simulink model "NMPC"  (R2017b)
settings: Solver=ode1  StartTime=0.0  StopTime=parSim.Tsim  FixedStep=0.001  RelTol=1e-3  EnableMultiTasking=on
values from neighbouring files (symbols this model uses):
  sysD_Delay = ss(A_Delay,B_Delay,C_Delay,D_Delay,parNMPC.Ts)    [main_GW02.m]
undefined symbols (not defined in the file or in its folder): parNMPC, parSim
libraries: simulink x1
settings Model: Creator=shaen  LastModifiedBy=severine

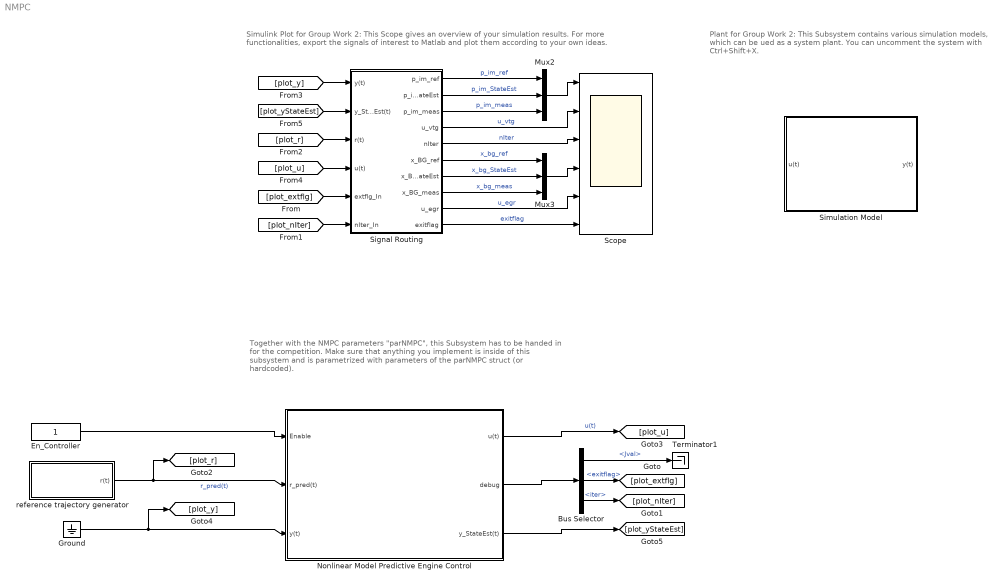
== system NMPC ==
  note: Plant for Group Work 2: This Subsystem contains various
      | simulation models, which can be ued as a system plant. You
      | can uncomment the system with Ctrl+Shift+X.
  note: Together with the NMPC parameters "parNMPC", this Subsystem
      | has to be handed in for the competition. Make sure that
      | anything you implement is inside of this subsystem and is
      | parametrized with parameters of the parNMPC struct (or
      | hardcoded).
  note: Simulink Plot for Group Work 2: This Scope gives an overview of your simulation results.
      | For more functionalities, export the signals of interest to Matlab and plot them according to your
      | own ideas.
  Bus Selector : BusSelector  OutputSignals=Jval,exitflag,iter
  En_Controller : Constant  OutDataTypeStr=boolean
  Ground : Ground
  Mux2 : Mux  Inputs=3
  Mux3 : Mux  Inputs=3
  Nonlinear Model Predictive Engine Control : Subsystem  Description=test
  Scope : Scope  NumInputPorts=6
  Signal Routing : Subsystem
  Simulation Model : Subsystem
  Terminator1 : Terminator
  reference trajectory generator : Subsystem  mask{N=parNMPC.N, Ts=parNMPC.Ts}
      mask prompts: N "NMPC Horizon"; Ts "NMPC Time Step"
      mask DialogControl DescGroupVar Prompt: Reference Generator
      mask DialogControl DescTextVar Prompt: Derivation of the reference vecotrs for every time step for a non-causal NMPC approach.
  wires:
  Signal Routing/10(exitflag) -> Scope/6  "exitflag"
  Mux3/1 -> Scope/4
  Nonlinear Model Predictive Engine Control/2(debug) -> Bus Selector/1
  [plot_r] -> Signal Routing/3(r(t))
  Signal Routing/5(nIter) -> Scope/3  "nIter"
  Signal Routing/4(u_vtg) -> Scope/2  "u_vtg"
  [plot_u] -> Signal Routing/4(u(t))
  Signal Routing/8(x_BG_meas) -> Mux3/3  "x_bg_meas"
  Signal Routing/6(x_BG_ref) -> Mux3/1  "x_bg_ref"
  Mux2/1 -> Scope/1
  Signal Routing/1(p_im_ref) -> Mux2/1  "p_im_ref"
  Bus Selector/3 -> [plot_nIter]  "<iter>"
  reference trajectory generator/1(r(t)) -> [plot_r], Nonlinear Model Predictive Engine Control/2(r_pred(t))  "r_pred(t)"
  Nonlinear Model Predictive Engine Control/1(u(t)) -> [plot_u]  "u(t)"
  Signal Routing/3(p_im_meas) -> Mux2/3  "p_im_meas"
  [plot_y] -> Signal Routing/1(y(t))
  [plot_extflg] -> Signal Routing/5(extflg_In)
  Signal Routing/9(u_egr) -> Scope/5  "u_egr"
  Bus Selector/1 -> Terminator1/1  "<Jval>"
  [plot_nIter] -> Signal Routing/6(nIter_In)
  Bus Selector/2 -> [plot_extflg]  "<exitflag>"
  Nonlinear Model Predictive Engine Control/3(y_StateEst(t)) -> [plot_yStateEst]
  [plot_yStateEst] -> Signal Routing/2(y_StateEst(t))
  Signal Routing/7(x_BG_StateEst) -> Mux3/2  "x_bg_StateEst"
  Signal Routing/2(p_im_StateEst) -> Mux2/2  "p_im_StateEst"
  En_Controller/1 -> Nonlinear Model Predictive Engine Control/1(Enable)
  Ground/1 -> [plot_y], Nonlinear Model Predictive Engine Control/3(y(t))

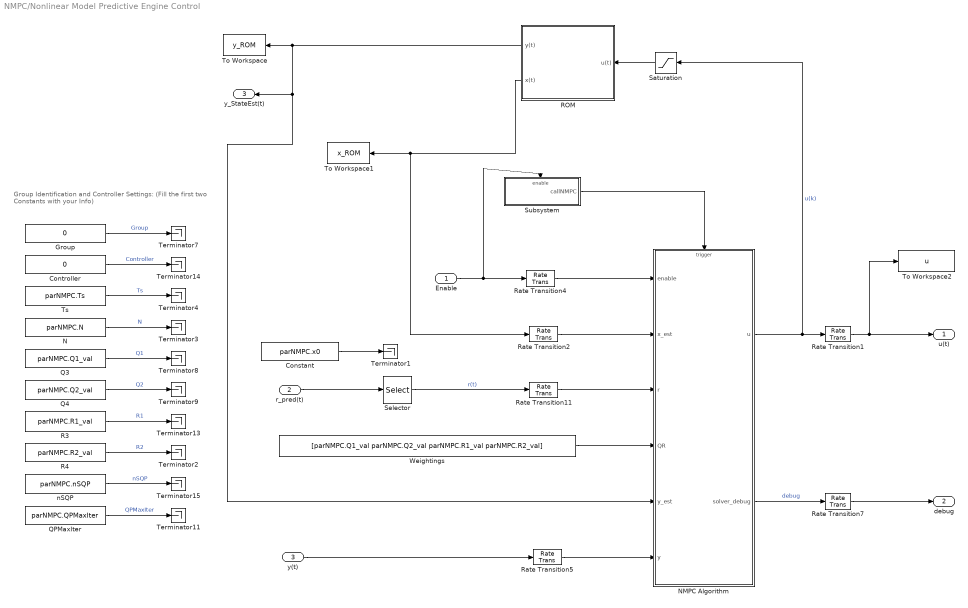
== system NMPC/Nonlinear Model Predictive Engine Control ==
  note: Group Identification and Controller Settings:
      | (Fill the first two Constants with your Info)
  Enable : Inport
  r_pred(t) : Inport  Port=2
  y(t) : Inport  Port=3
  Constant : Constant  Value=parNMPC.x0
  Controller : Constant  Value=0
  Group : Constant  Value=0
  N : Constant  Value=parNMPC.N
  NMPC Algorithm : Subsystem
  Q3 : Constant  Value=parNMPC.Q1_val
  Q4 : Constant  Value=parNMPC.Q2_val
  QPMaxIter : Constant  Value=parNMPC.QPMaxIter
  R3 : Constant  Value=parNMPC.R1_val
  R4 : Constant  Value=parNMPC.R2_val
  ROM : Subsystem  TreatAsAtomicUnit=on
  Rate Transition1 : RateTransition
  Rate Transition11 : RateTransition  InitialCondition=parNMPC.y0
  Rate Transition2 : RateTransition  InitialCondition=parNMPC.x0
  Rate Transition4 : RateTransition
  Rate Transition5 : RateTransition  InitialCondition=parNMPC.y0
  Rate Transition7 : RateTransition
  Saturation : Saturate  UpperLimit=Inf  LowerLimit=-Inf
  Selector : Selector  InputPortWidth=parNMPC.N*parNMPC.nOutputs  IndexOptions=Index vector (dialog)  Indices=[1,parNMPC.N+1]  OutputSizes=1
  Subsystem : Subsystem
  Terminator{1..4,7..9,11,13..15} (11 alike) : Terminator
  To Workspace : ToWorkspace  VariableName=y_ROM  SaveFormat=Timeseries  SampleTime=-1
  To Workspace1 : ToWorkspace  VariableName=x_ROM  SaveFormat=Timeseries  SampleTime=-1
  To Workspace2 : ToWorkspace  VariableName=u  SaveFormat=Timeseries  SampleTime=-1
  Ts : Constant  Value=parNMPC.Ts
  Weightings : Constant  Value=[parNMPC.Q1_val parNMPC.Q2_val parNMPC.R1_val parNMPC.R2_val]
  nSQP : Constant  Value=parNMPC.nSQP
  u(t) : Outport
  debug : Outport  Port=2
  y_StateEst(t) : Outport  Port=3
  wires:
  R4/1 -> Terminator2/1  "R2"
  Ts/1 -> Terminator4/1  "Ts"
  nSQP/1 -> Terminator15/1  "nSQP"
  R3/1 -> Terminator13/1  "R1"
  Q3/1 -> Terminator8/1  "Q1"
  N/1 -> Terminator3/1  "N"
  Group/1 -> Terminator7/1  "Group"
  QPMaxIter/1 -> Terminator11/1  "QPMaxIter"
  Controller/1 -> Terminator14/1  "Controller"
  Q4/1 -> Terminator9/1  "Q2"
  Selector/1 -> Rate Transition11/1  "r(t)"
  r_pred(t)/1 -> Selector/1
  Rate Transition7/1 -> debug/1
  NMPC Algorithm/1(u) -> Saturation/1, Rate Transition1/1  "u(k)"
  y(t)/1 -> Rate Transition5/1
  NMPC Algorithm/2(solver_debug) -> Rate Transition7/1  "debug"
  Rate Transition2/1 -> NMPC Algorithm/2("x_est ")
  Rate Transition1/1 -> u(t)/1, To Workspace2/1
  Enable/1 -> Subsystem/Enable, Rate Transition4/1
  Rate Transition4/1 -> NMPC Algorithm/1(enable)
  Subsystem/1(callNMPC) -> NMPC Algorithm/Trigger
  Rate Transition5/1 -> NMPC Algorithm/6(y)
  Rate Transition11/1 -> NMPC Algorithm/3(r)
  Weightings/1 -> NMPC Algorithm/4(QR)
  Constant/1 -> Terminator1/1
  ROM/1(y(t)) -> NMPC Algorithm/5(y_est), y_StateEst(t)/1, To Workspace/1
  ROM/2(x(t)) -> Rate Transition2/1, To Workspace1/1
  Saturation/1 -> ROM/1(u(t))

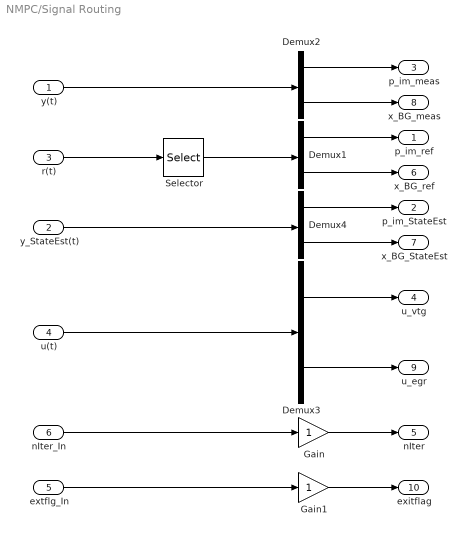
== system NMPC/Signal Routing ==
  y(t) : Inport
  y_StateEst(t) : Inport  Port=2
  r(t) : Inport  Port=3
  u(t) : Inport  Port=4
  extflg_In : Inport  Port=5
  nIter_In : Inport  Port=6
  Demux{1..4} (4 alike) : Demux  Outputs=2
  Gain : Gain
  Gain1 : Gain
  Selector : Selector  InputPortWidth=parNMPC.N*parNMPC.nOutputs  IndexOptions=Index vector (dialog)  Indices=[1,parNMPC.N+1]  OutputSizes=1
  p_im_ref : Outport
  p_im_StateEst : Outport  Port=2
  p_im_meas : Outport  Port=3
  u_vtg : Outport  Port=4
  nIter : Outport  Port=5
  x_BG_ref : Outport  Port=6
  x_BG_StateEst : Outport  Port=7
  x_BG_meas : Outport  Port=8
  u_egr : Outport  Port=9
  exitflag : Outport  Port=10
  wires:
  nIter_In/1 -> Gain/1
  Demux2/2 -> x_BG_meas/1
  Demux1/1 -> p_im_ref/1
  Demux3/2 -> u_egr/1
  extflg_In/1 -> Gain1/1
  y(t)/1 -> Demux2/1
  r(t)/1 -> Selector/1
  Demux1/2 -> x_BG_ref/1
  u(t)/1 -> Demux3/1
  Demux3/1 -> u_vtg/1
  Demux2/1 -> p_im_meas/1
  Selector/1 -> Demux1/1
  y_StateEst(t)/1 -> Demux4/1
  Demux4/2 -> x_BG_StateEst/1
  Demux4/1 -> p_im_StateEst/1
  Gain/1 -> nIter/1
  Gain1/1 -> exitflag/1

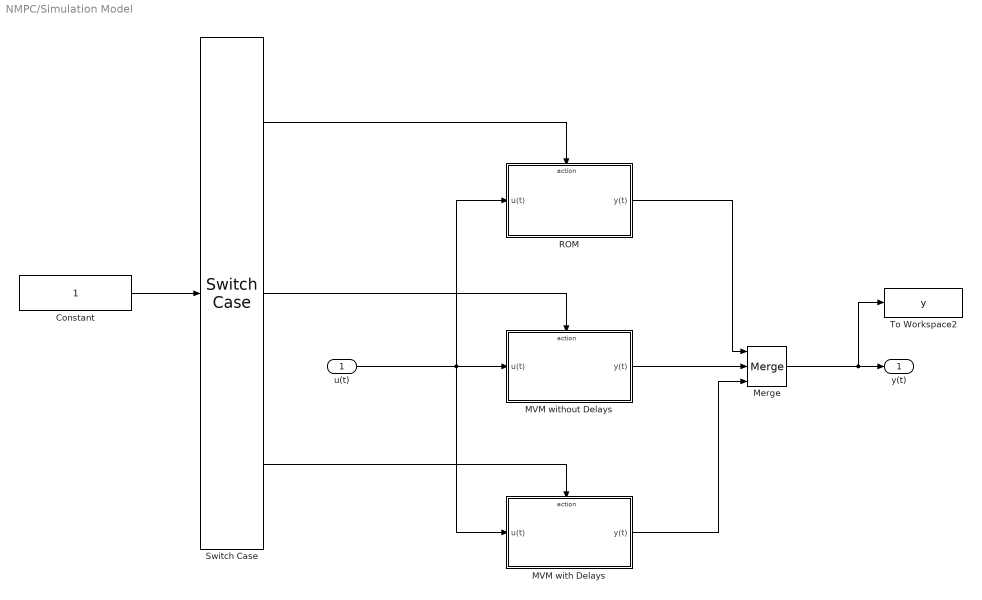
== system NMPC/Simulation Model ==
  u(t) : Inport
  Constant : Constant
  MVM with Delays : Subsystem  TreatAsAtomicUnit=on
  MVM without Delays : Subsystem  TreatAsAtomicUnit=on
  Merge : Merge  Inputs=3
  ROM : Subsystem  TreatAsAtomicUnit=on
  Switch Case : SwitchCase  CaseConditions={1,2,3}  ShowDefaultCase=off
  To Workspace2 : ToWorkspace  VariableName=y  SaveFormat=Timeseries  SampleTime=-1
  y(t) : Outport
  wires:
  u(t)/1 -> MVM with Delays/1(u(t)), ROM/1(u(t)), MVM without Delays/1(u(t))
  Constant/1 -> Switch Case/1
  MVM without Delays/1(y(t)) -> Merge/2
  Merge/1 -> To Workspace2/1, y(t)/1
  MVM with Delays/1(y(t)) -> Merge/3
  Switch Case/2 -> MVM without Delays/Action
  Switch Case/3 -> MVM with Delays/Action
  Switch Case/1 -> ROM/Action
  ROM/1(y(t)) -> Merge/1

== system NMPC/reference trajectory generator ==
  1-D Lookup Table : Lookup_n-D  NumberOfTableDimensions=1  BreakpointsForDimension1=parSim.ref.p_im.time  Table=parSim.ref.p_im.data  ExtrapMethod=Clip  InternalRulePriority=Speed  RndMeth=Simplest  InputSameDT=on
  1-D Lookup Table1 : Lookup_n-D  NumberOfTableDimensions=1  BreakpointsForDimension1=parSim.ref.x_bg.time  Table=parSim.ref.x_bg.data  InternalRulePriority=Speed  RndMeth=Simplest  InputSameDT=on
  Clock : Clock
  MATLAB Function : MATLAB Function  TreatAsAtomicUnit=on
  Mux : Mux  Inputs=2
  r(t) : Outport
  wires:
  MATLAB Function/1(y) -> 1-D Lookup Table1/1, 1-D Lookup Table/1
  1-D Lookup Table/1 -> Mux/1
  1-D Lookup Table1/1 -> Mux/2
  Mux/1 -> r(t)/1
  Clock/1 -> MATLAB Function/1(u)  "refTime"

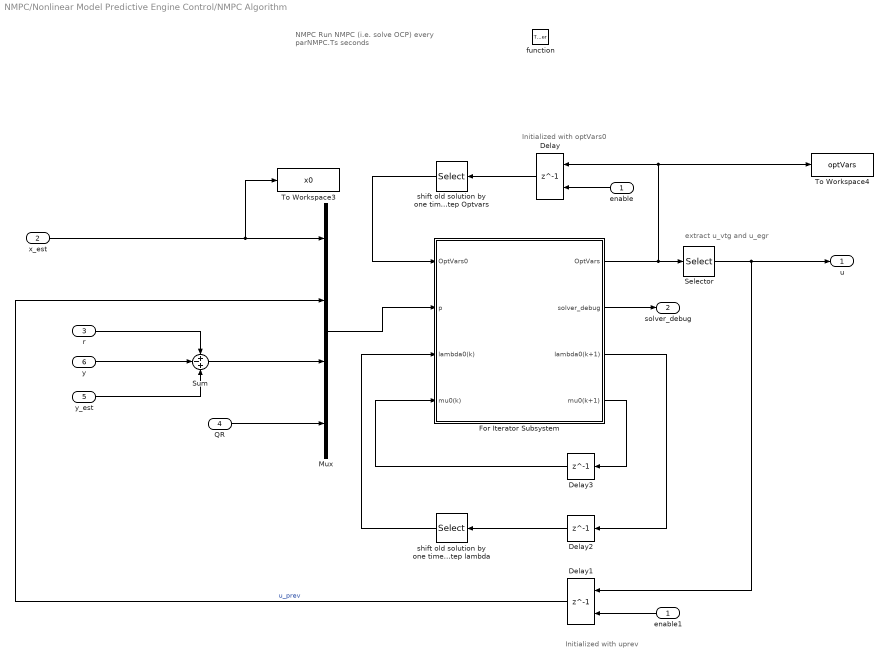
== system NMPC/Nonlinear Model Predictive Engine Control/NMPC Algorithm ==
  note: extract u_vtg and u_egr
  note: Initialized with uprev
  note: NMPC
      | Run NMPC (i.e. solve OCP) every parNMPC.Ts seconds
  note: Initialized with optVars0
  enable : Inport
  "x_est " : Inport  Port=2
  r : Inport  Port=3
  QR : Inport  Port=4
  y_est : Inport  Port=5
  y : Inport  Port=6
  function : TriggerPort  TriggerType=function-call  VariantControl=Variant  SampleTimeType=periodic  SampleTime=-1
  Delay : Delay  DelayLength=1  InitialCondition=parNMPC.optVars0  ExternalReset=Rising
      settings: InputPortMap=u0,r5
  Delay1 : Delay  DelayLength=1  InitialCondition=parNMPC.uprev  ExternalReset=Rising
      settings: InputPortMap=u0,r5
  Delay2 : Delay  DelayLength=1  InitialCondition=parNMPC.lambda0
  Delay3 : Delay  DelayLength=1  InitialCondition=parNMPC.mu0
  For Iterator Subsystem : Subsystem  TreatAsAtomicUnit=on
  Mux : Mux
  Selector : Selector  InputPortWidth=parNMPC.nOptVars  IndexOptions=Index vector (dialog)  Indices=[1,2]  OutputSizes=1
  Sum : Sum  Inputs=+-+
  To Workspace3 : ToWorkspace  VariableName=x0  SaveFormat=Timeseries  SampleTime=-1
  To Workspace4 : ToWorkspace  VariableName=optVars  SaveFormat=Timeseries  SampleTime=-1
  enable1 : InportShadow
  shift old solution by one timestep Optvars : Selector  InputPortWidth=parNMPC.nOptVars  IndexOptions=Index vector (dialog)  Indices=[(parNMPC.nInputs+parNMPC.nStates+1):parNMPC.nOptVars, parNMPC.nOptVars-(parNMPC.nInputs+parNMPC.nStates-1):parNMPC.nOptVars]  OutputSizes=1
  shift old solution by one timestep lambda : Selector  InputPortWidth=parNMPC.nConstr  IndexOptions=Index vector (dialog)  Indices=[(parNMPC.nStates+1):parNMPC.nConstr, parNMPC.nConstr-(parNMPC.nStates-1):parNMPC.nConstr]  OutputSizes=1
  u : Outport  InitialOutput=parNMPC.uprev
  solver_debug : Outport  Port=2
  wires:
  For Iterator Subsystem/2(solver_debug) -> solver_debug/1
  Selector/1 -> u/1, Delay1/1
  enable/1 -> Delay/2
  "x_est "/1 -> Mux/1, To Workspace3/1
  For Iterator Subsystem/3(lambda0(k+1)) -> Delay2/1
  Delay/1 -> shift old solution by one timestep Optvars/1
  QR/1 -> Mux/4
  Delay3/1 -> For Iterator Subsystem/4(mu0(k))
  shift old solution by one timestep Optvars/1 -> For Iterator Subsystem/1(OptVars0)
  Delay2/1 -> shift old solution by one timestep lambda/1
  For Iterator Subsystem/1(OptVars) -> Selector/1, To Workspace4/1, Delay/1
  shift old solution by one timestep lambda/1 -> For Iterator Subsystem/3(lambda0(k))
  For Iterator Subsystem/4(mu0(k+1)) -> Delay3/1
  Delay1/1 -> Mux/2  "u_prev"
  enable1/1 -> Delay1/2
  Mux/1 -> For Iterator Subsystem/2(p)
  y_est/1 -> Sum/3
  y/1 -> Sum/2
  r/1 -> Sum/1
  Sum/1 -> Mux/3

== system NMPC/Nonlinear Model Predictive Engine Control/ROM ==
  u(t) : Inport
  ROM : Subsystem
  Saturation1 : Saturate  UpperLimit=1  LowerLimit=0
  Terminator1 : Terminator
  y(t) : Outport
  x(t) : Outport  Port=2
  wires:
  u(t)/1 -> Saturation1/1
  ROM/1(y) -> y(t)/1
  Saturation1/1 -> ROM/1(u)
  ROM/2(x) -> Terminator1/1, x(t)/1

== system NMPC/Nonlinear Model Predictive Engine Control/Subsystem ==
  Enable1 : EnablePort
  Function-Call Generator : simulink/Ports & Subsystems/Function-Call Generator  sample_time=parNMPC.Ts  numberOfIterations=1
  callNMPC : Outport
  wires:
  Function-Call Generator/1 -> callNMPC/1

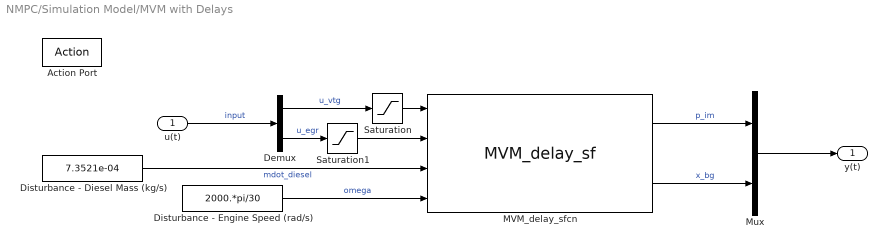
== system NMPC/Simulation Model/MVM with Delays ==
  u(t) : Inport
  Action Port : ActionPort  ActionType=case
  Demux : Demux  Outputs=2
  Disturbance - Diesel Mass (kg/s) : Constant  Value=7.3521e-04
  Disturbance - Engine Speed (rad/s) : Constant  Value=2000.*pi/30
  MVM_delay_sfcn : S-Function  FunctionName=MVM_delay_sf  SFunctionModules=""  SFunctionDeploymentMode=off  EnableBusSupport=off  SFcnStateName=DWORK0  mask{rtw_sf_name=MVM_delay_sf, showVar=off}
      mask prompts: rtw_sf_name "Simulink:masks:GenSFuncName_MP"; showVar "Simulink:masks:GenSFuncShowModuleList_MP"
      mask help: Simulink:masks:GenSFuncDesc_MD
      mask init:
      | displist = '';
      | if ~strcmp(get_param(gcb, 'FunctionName'), rtw_sf_name);
      |   set_param(gcb, 'FunctionName', rtw_sf_name);
      | end
      | % Check if we are generating code
      | rtw_mode = false;
      | if strcmpi(get_param(bdroot(gcb),'SimulationStatus'),'Initializing')
      | 	rtw_mode = strcmpi(get_param(bdroot(gcb),'BuildingRTWCode'),'on') && ...
      | 		~strcmpi(get_param(bdroot(gcb),'TargetStyle'),'SimulationTarget');
      | end
      | if showVar || rtw_mode
      | 	if exist('rtwsfunc') == 2 | exist('rtwsfunc') == 6
      | 		tmplist = rtwsfunc(rtw_sf_name,gcb);
      | 		tmplist = DAStudio.message('Simulink:masks:GenSFuncListOfModules_IC', tmplist);
      | 	elseif showVar
      | 		tmplist1 = DAStudio.message('Simulink:masks:GenSFuncListOfModules_IC', '');
      |         tmplist2 = DAStudio.message('Simulink:masks:GenSFuncNotLicensed_IC');
      |         tmplist = [tmplist1 tmplist2];
      |  	end
      | end
      | if showVar
      |   displist = tmplist;
      | end
      settings: SFcnIsStateOwnerBlock=on
      settings: CopyFcn=|
      | if ~strcmp(get_param(gcb,'Linkstatus'),'none') && ...
      | ~strcmp(get_param(gcb,'Linkstatus'),'implicit')
      |   set_param(gcb,'LinkStatus','none');
      | end
      mask Help: eval('feval(''rtwprivate'',''rtwhelpview'',''rtw_sfcn_block'')');
      mask Display:
      | port_label('input',1,'u_vtg');
      | port_label('input',2,'u_egr');
      | port_label('input',3,'mdot_diesel');
      | port_label('input',4,'omega');
      | port_label('output',1,'p_im');
      | port_label('output',2,'x_bg');
  Mux : Mux  Inputs=2
  Saturation : Saturate  UpperLimit=1  LowerLimit=0
  Saturation1 : Saturate  UpperLimit=1  LowerLimit=0
  y(t) : Outport
  wires:
  Saturation/1 -> MVM_delay_sfcn/1
  Disturbance - Engine Speed (rad/s)/1 -> MVM_delay_sfcn/4  "omega"
  Mux/1 -> y(t)/1
  u(t)/1 -> Demux/1  "input"
  MVM_delay_sfcn/1 -> Mux/1  "p_im"
  Saturation1/1 -> MVM_delay_sfcn/2
  Disturbance - Diesel Mass (kg/s)/1 -> MVM_delay_sfcn/3  "mdot_diesel"
  MVM_delay_sfcn/2 -> Mux/2  "x_bg"
  Demux/2 -> Saturation1/1  "u_egr"
  Demux/1 -> Saturation/1  "u_vtg"

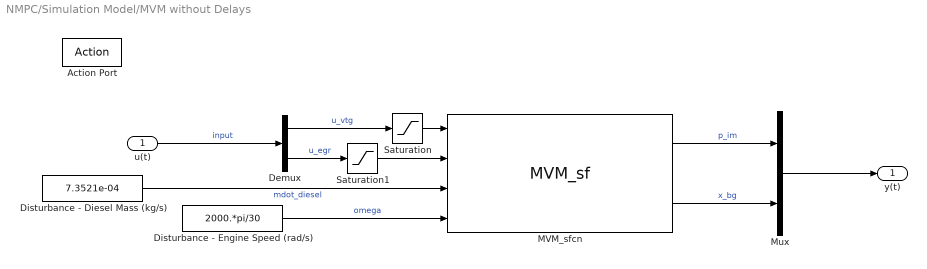
== system NMPC/Simulation Model/MVM without Delays ==
  u(t) : Inport
  Action Port : ActionPort  ActionType=case
  Demux : Demux  Outputs=2
  Disturbance - Diesel Mass (kg/s) : Constant  Value=7.3521e-04
  Disturbance - Engine Speed (rad/s) : Constant  Value=2000.*pi/30
  MVM_sfcn : S-Function  FunctionName=MVM_sf  SFunctionModules=""  SFunctionDeploymentMode=off  EnableBusSupport=off  SFcnStateName=DWORK0  mask{rtw_sf_name=MVM_sf, showVar=off}
      mask prompts: rtw_sf_name "Simulink:masks:GenSFuncName_MP"; showVar "Simulink:masks:GenSFuncShowModuleList_MP"
      mask help: Simulink:masks:GenSFuncDesc_MD
      mask init: same as NMPC/Simulation Model/MVM with Delays/MVM_delay_sfcn
      settings: SFcnIsStateOwnerBlock=on
      settings: CopyFcn=|
      | if ~strcmp(get_param(gcb,'Linkstatus'),'none') && ...
      | ~strcmp(get_param(gcb,'Linkstatus'),'implicit')
      |   set_param(gcb,'LinkStatus','none');
      | end
      mask Help: eval('feval(''rtwprivate'',''rtwhelpview'',''rtw_sfcn_block'')');
      mask Display:
      | port_label('input',1,'u_vtg');
      | port_label('input',2,'u_egr');
      | port_label('input',3,'mdot_diesel');
      | port_label('input',4,'omega');
      | port_label('output',1,'p_im');
      | port_label('output',2,'x_bg');
  Mux : Mux  Inputs=2
  Saturation : Saturate  UpperLimit=1  LowerLimit=0
  Saturation1 : Saturate  UpperLimit=1  LowerLimit=0
  y(t) : Outport
  wires:
  Mux/1 -> y(t)/1
  MVM_sfcn/2 -> Mux/2  "x_bg"
  u(t)/1 -> Demux/1  "input"
  Disturbance - Diesel Mass (kg/s)/1 -> MVM_sfcn/3  "mdot_diesel"
  Demux/1 -> Saturation/1  "u_vtg"
  Demux/2 -> Saturation1/1  "u_egr"
  Disturbance - Engine Speed (rad/s)/1 -> MVM_sfcn/4  "omega"
  MVM_sfcn/1 -> Mux/1  "p_im"
  Saturation1/1 -> MVM_sfcn/2
  Saturation/1 -> MVM_sfcn/1

== system NMPC/Simulation Model/ROM ==
  u(t) : Inport
  Action Port : ActionPort  ActionType=case
  ROM : Subsystem
  Saturation1 : Saturate  UpperLimit=1  LowerLimit=0
  Terminator1 : Terminator
  y(t) : Outport
  wires:
  ROM/2(x) -> Terminator1/1
  Saturation1/1 -> ROM/1(u)
  u(t)/1 -> Saturation1/1
  ROM/1(y) -> y(t)/1

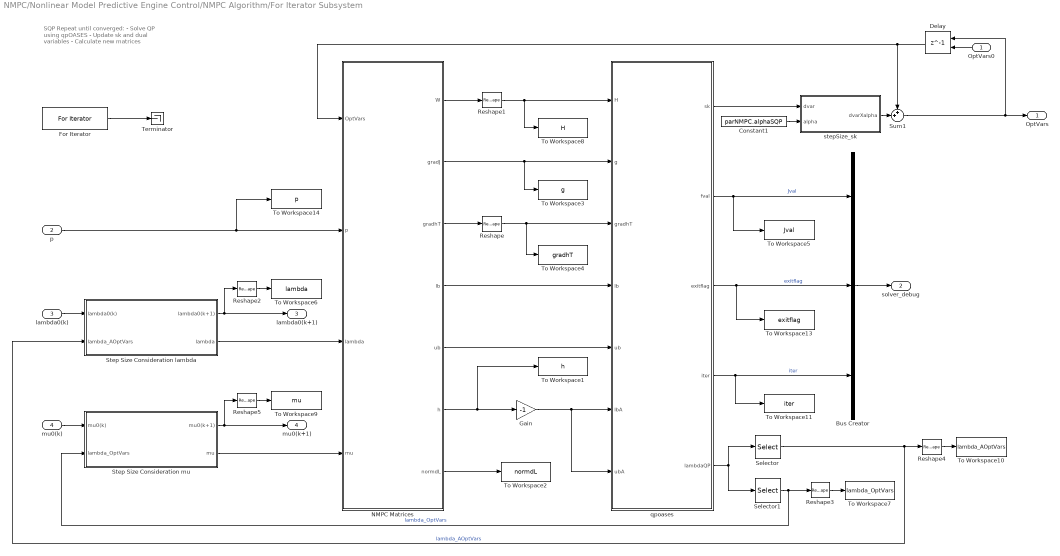
== system NMPC/Nonlinear Model Predictive Engine Control/NMPC Algorithm/For Iterator Subsystem ==
  note: SQP
      | Repeat until converged:
      | - Solve QP using qpOASES
      | - Update sk and dual variables
      | - Calculate new matrices
  OptVars0 : Inport
  p : Inport  Port=2
  lambda0(k) : Inport  Port=3
  mu0(k) : Inport  Port=4
  Bus Creator : BusCreator  Inputs=3
  Constant1 : Constant  Value=parNMPC.alphaSQP
  Delay : Delay  DelayLength=1  InitialConditionSource=Input port  InitialCondition=0
      settings: InputPortMap=u0,p4
  For Iterator : ForIterator  ResetStates=reset  IterationLimit=parNMPC.nSQP
  Gain : Gain  Gain=-1
  NMPC Matrices : Subsystem
  Reshape{,1..5} (6 alike) : Reshape  OutputDimensionality=Column vector (2-D)
  Selector : Selector  InputPortWidth=parNMPC.nOptVars+parNMPC.nConstr  IndexOptions=Index vector (dialog)  Indices=[parNMPC.nOptVars+1:parNMPC.nOptVars+parNMPC.nConstr]  OutputSizes=1
  Selector1 : Selector  InputPortWidth=parNMPC.nOptVars+parNMPC.nConstr  IndexOptions=Index vector (dialog)  Indices=[1:parNMPC.nOptVars]  OutputSizes=1
  Step Size Consideration lambda : Subsystem
  Step Size Consideration mu : Subsystem
  Sum1 : Sum  Inputs=++|
  Terminator : Terminator
  To Workspace1 : ToWorkspace  VariableName=h  SaveFormat=Timeseries  SampleTime=-1
  To Workspace10 : ToWorkspace  VariableName=lambda_AOptVars  SaveFormat=Timeseries  SampleTime=-1
  To Workspace11 : ToWorkspace  VariableName=iter  SaveFormat=Timeseries  SampleTime=-1
  To Workspace13 : ToWorkspace  VariableName=exitflag  SaveFormat=Timeseries  SampleTime=-1
  To Workspace14 : ToWorkspace  VariableName=p  SaveFormat=Timeseries  SampleTime=-1
  To Workspace2 : ToWorkspace  VariableName=normdL  SaveFormat=Timeseries  SampleTime=-1
  To Workspace3 : ToWorkspace  VariableName=g  SaveFormat=Timeseries  SampleTime=-1
  To Workspace4 : ToWorkspace  VariableName=gradhT  SaveFormat=Timeseries  SampleTime=-1
  To Workspace5 : ToWorkspace  VariableName=Jval  SaveFormat=Timeseries  SampleTime=-1
  To Workspace6 : ToWorkspace  VariableName=lambda  SaveFormat=Timeseries  SampleTime=-1
  To Workspace7 : ToWorkspace  VariableName=lambda_OptVars  SaveFormat=Timeseries  SampleTime=-1
  To Workspace8 : ToWorkspace  VariableName=H  SaveFormat=Timeseries  SampleTime=-1
  To Workspace9 : ToWorkspace  VariableName=mu  SaveFormat=Timeseries  SampleTime=-1
  qpoases : Subsystem
  stepSize_sk : MATLAB Function  TreatAsAtomicUnit=on
  OptVars : Outport
  solver_debug : Outport  Port=2
  lambda0(k+1) : Outport  Port=3
  mu0(k+1) : Outport  Port=4
  wires:
  Bus Creator/1 -> solver_debug/1
  Reshape/1 -> To Workspace4/1, qpoases/3(gradhT)
  Gain/1 -> qpoases/7(ubA), qpoases/6(lbA)
  Delay/1 -> Sum1/1, NMPC Matrices/1(OptVars)
  Sum1/1 -> OptVars/1, Delay/1
  OptVars0/1 -> Delay/2
  qpoases/4(iter) -> Bus Creator/3, To Workspace11/1  "iter"
  NMPC Matrices/5(ub) -> qpoases/5(ub)
  NMPC Matrices/4(lb) -> qpoases/4(lb)
  NMPC Matrices/3(gradhT) -> Reshape/1
  qpoases/2(fval) -> Bus Creator/1, To Workspace5/1  "Jval"
  Reshape1/1 -> qpoases/1(H), To Workspace8/1
  NMPC Matrices/1(W) -> Reshape1/1
  NMPC Matrices/2(gradJ) -> qpoases/2(g), To Workspace3/1
  qpoases/3(exitflag) -> Bus Creator/2, To Workspace13/1  "exitflag"
  NMPC Matrices/6(h) -> To Workspace1/1, Gain/1
  p/1 -> NMPC Matrices/2(p), To Workspace14/1
  qpoases/1(sk) -> stepSize_sk/1(dvar)
  stepSize_sk/1(dvarXalpha) -> Sum1/2
  NMPC Matrices/7(normdL) -> To Workspace2/1
  For Iterator/1 -> Terminator/1
  mu0(k)/1 -> Step Size Consideration mu/1(mu0(k))
  qpoases/5(lambdaQP) -> Selector/1, Selector1/1
  Step Size Consideration lambda/2(lambda) -> NMPC Matrices/3(lambda)
  Step Size Consideration mu/2(mu) -> NMPC Matrices/4(mu)
  Step Size Consideration mu/1(mu0(k+1)) -> Reshape5/1, mu0(k+1)/1
  Reshape5/1 -> To Workspace9/1
  Reshape2/1 -> To Workspace6/1
  Step Size Consideration lambda/1(lambda0(k+1)) -> lambda0(k+1)/1, Reshape2/1
  lambda0(k)/1 -> Step Size Consideration lambda/1(lambda0(k))
  Selector1/1 -> Step Size Consideration mu/2(lambda_OptVars), Reshape3/1  "lambda_OptVars"
  Selector/1 -> Reshape4/1, Step Size Consideration lambda/2(lambda_AOptVars)  "lambda_AOptVars"
  Reshape3/1 -> To Workspace7/1
  Reshape4/1 -> To Workspace10/1
  Constant1/1 -> stepSize_sk/2(alpha)

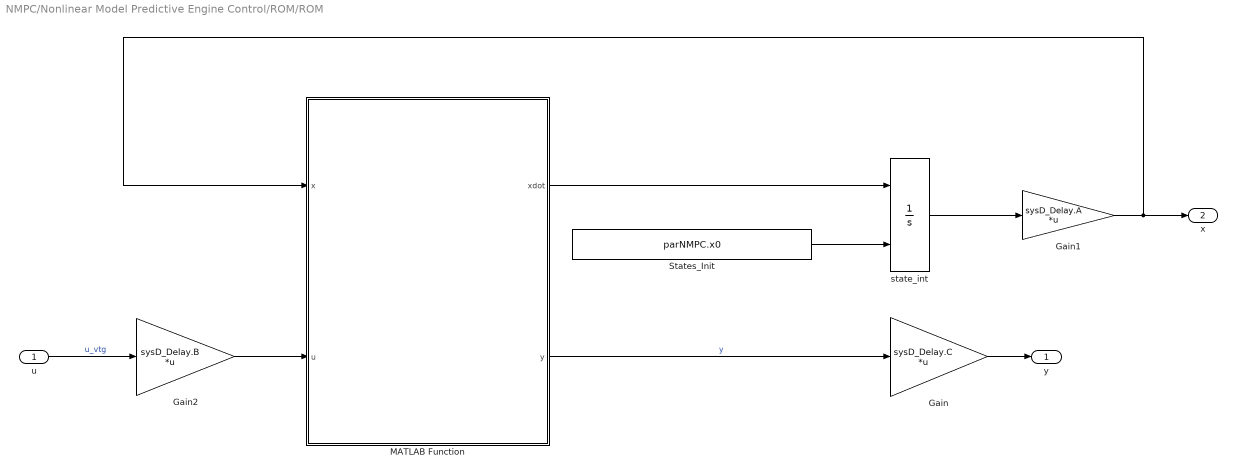
== system NMPC/Nonlinear Model Predictive Engine Control/ROM/ROM ==
  u : Inport
  Gain : Gain  Gain=sysD_Delay.C  Multiplication=Matrix(K*u)
  Gain1 : Gain  Gain=sysD_Delay.A  Multiplication=Matrix(K*u)
  Gain2 : Gain  Gain=sysD_Delay.B  Multiplication=Matrix(K*u)
  MATLAB Function : MATLAB Function  TreatAsAtomicUnit=on
  States_Init : Constant  Value=parNMPC.x0
  state_int : Integrator  InitialConditionSource=external  InitialCondition=0.55  ContinuousStateAttributes=['n_tc' 'p_im' 'p_em' 'F_im' 'F_em']
  y : Outport  Tag=p_im
  x : Outport  Port=2
  wires:
  MATLAB Function/1(xdot) -> state_int/1
  States_Init/1 -> state_int/2
  Gain2/1 -> MATLAB Function/2(u)
  u/1 -> Gain2/1  "u_vtg"
  Gain/1 -> y/1
  MATLAB Function/2(y) -> Gain/1  "y"
  state_int/1 -> Gain1/1
  Gain1/1 -> MATLAB Function/1(x), x/1

== system NMPC/Simulation Model/ROM/ROM ==
  u : Inport
  MATLAB Function : MATLAB Function  TreatAsAtomicUnit=on
  States_Init : Constant  Value=parNMPC.x0
  state_int : Integrator  InitialConditionSource=external  InitialCondition=0.55  ContinuousStateAttributes=['n_tc' 'p_im' 'p_em' 'F_im' 'F_em']
  y : Outport  Tag=p_im
  x : Outport  Port=2
  wires:
  MATLAB Function/1(xdot) -> state_int/1
  u/1 -> MATLAB Function/2(u)  "u_vtg"
  MATLAB Function/2(y) -> y/1  "y"
  state_int/1 -> MATLAB Function/1(x), x/1
  States_Init/1 -> state_int/2

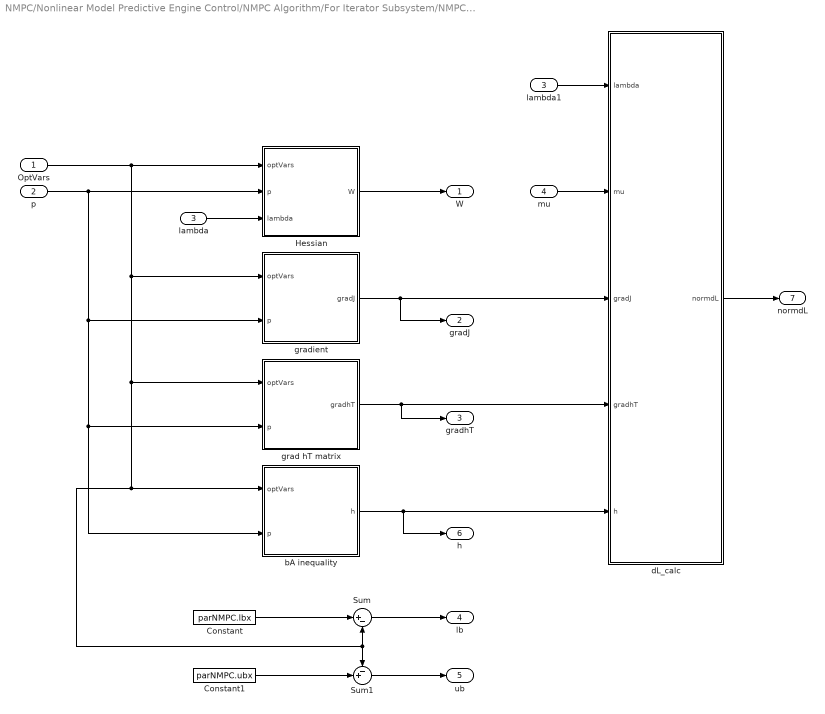
== system NMPC/Nonlinear Model Predictive Engine Control/NMPC Algorithm/For Iterator Subsystem/NMPC Matrices ==
  OptVars : Inport
  p : Inport  Port=2
  lambda : Inport  Port=3
  mu : Inport  Port=4
  Constant : Constant  Value=parNMPC.lbx
  Constant1 : Constant  Value=parNMPC.ubx
  Hessian : Subsystem
  Sum : Sum  Inputs=|+-
  Sum1 : Sum  Inputs=-+|
  bA inequality : Subsystem
  dL_calc : MATLAB Function  TreatAsAtomicUnit=on
  grad hT matrix : Subsystem
  gradient : Subsystem
  lambda1 : InportShadow  Port=3
  W : Outport
  gradJ : Outport  Port=2
  gradhT : Outport  Port=3
  lb : Outport  Port=4
  ub : Outport  Port=5
  h : Outport  Port=6
  normdL : Outport  Port=7
  wires:
  Sum1/1 -> ub/1
  Sum/1 -> lb/1
  p/1 -> bA inequality/2(p), grad hT matrix/2(p), gradient/2(p), Hessian/2(p)
  bA inequality/1(h) -> h/1, dL_calc/5(h)
  grad hT matrix/1(gradhT) -> gradhT/1, dL_calc/4(gradhT)
  Hessian/1(W) -> W/1
  OptVars/1 -> Sum1/1, Sum/2, bA inequality/1(optVars), grad hT matrix/1(optVars), gradient/1(optVars), Hessian/1(optVars)
  gradient/1(gradJ) -> gradJ/1, dL_calc/3(gradJ)
  lambda/1 -> Hessian/3(lambda)
  lambda1/1 -> dL_calc/1(lambda)
  dL_calc/1(normdL) -> normdL/1
  mu/1 -> dL_calc/2(mu)
  Constant/1 -> Sum/1
  Constant1/1 -> Sum1/2

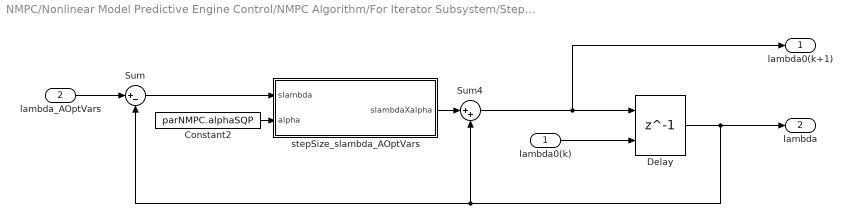
== system NMPC/Nonlinear Model Predictive Engine Control/NMPC Algorithm/For Iterator Subsystem/Step Size Consideration lambda ==
  lambda0(k) : Inport
  lambda_AOptVars : Inport  Port=2
  Constant2 : Constant  Value=parNMPC.alphaSQP
  Delay : Delay  DelayLength=1  InitialConditionSource=Input port  InitialCondition=0  UseCircularBuffer=on
      settings: InputPortMap=u0,p4
  Sum : Sum  Inputs=|+-
  Sum4 : Sum  Inputs=|++
  stepSize_slambda_AOptVars : MATLAB Function  TreatAsAtomicUnit=on
  lambda0(k+1) : Outport
  lambda : Outport  Port=2
  wires:
  lambda_AOptVars/1 -> Sum/1
  stepSize_slambda_AOptVars/1(slambdaXalpha) -> Sum4/1
  Sum/1 -> stepSize_slambda_AOptVars/1(slambda)
  Sum4/1 -> lambda0(k+1)/1, Delay/1
  lambda0(k)/1 -> Delay/2
  Delay/1 -> Sum4/2, Sum/2, lambda/1
  Constant2/1 -> stepSize_slambda_AOptVars/2(alpha)

== system NMPC/Nonlinear Model Predictive Engine Control/NMPC Algorithm/For Iterator Subsystem/Step Size Consideration mu ==
  mu0(k) : Inport
  lambda_OptVars : Inport  Port=2
  Constant3 : Constant  Value=parNMPC.alphaSQP
  Delay : Delay  DelayLength=1  InitialConditionSource=Input port  InitialCondition=0  UseCircularBuffer=on
      settings: InputPortMap=u0,p4
  Sum : Sum  Inputs=|+-
  Sum4 : Sum  Inputs=|++
  stepSize_slambda_OptVars : MATLAB Function  TreatAsAtomicUnit=on
  mu0(k+1) : Outport
  mu : Outport  Port=2
  wires:
  Delay/1 -> mu/1, Sum/2, Sum4/2
  mu0(k)/1 -> Delay/2
  Sum4/1 -> Delay/1, mu0(k+1)/1
  Sum/1 -> stepSize_slambda_OptVars/1(smu)
  stepSize_slambda_OptVars/1(smuXalpha) -> Sum4/1
  lambda_OptVars/1 -> Sum/1
  Constant3/1 -> stepSize_slambda_OptVars/2(alpha)

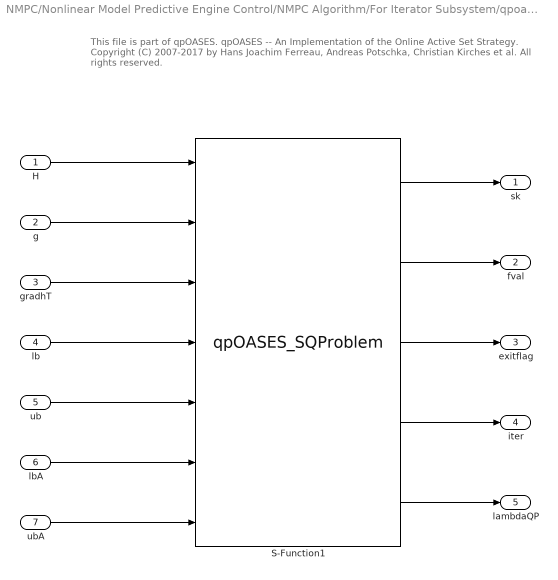
== system NMPC/Nonlinear Model Predictive Engine Control/NMPC Algorithm/For Iterator Subsystem/qpoases ==
  note: This file is part of qpOASES.
      |
      | qpOASES -- An Implementation of the Online Active Set Strategy.
      | Copyright (C) 2007-2017 by Hans Joachim Ferreau, Andreas Potschka, Christian Kirches et al.
      | All rights reserved.
  H : Inport
  g : Inport  Port=2
  gradhT : Inport  Port=3
  lb : Inport  Port=4
  ub : Inport  Port=5
  lbA : Inport  Port=6
  ubA : Inport  Port=7
  S-Function1 : S-Function  FunctionName=qpOASES_SQProblem  Parameters=parNMPC.nOptVars, parNMPC.QPMaxIter, parNMPC.nOptVars+parNMPC.nConstr  SFunctionDeploymentMode=off  EnableBusSupport=off
  sk : Outport
  fval : Outport  Port=2
  exitflag : Outport  Port=3
  iter : Outport  Port=4
  lambdaQP : Outport  Port=5
  wires:
  S-Function1/3 -> exitflag/1
  S-Function1/4 -> iter/1
  S-Function1/2 -> fval/1
  S-Function1/1 -> sk/1
  g/1 -> S-Function1/2
  H/1 -> S-Function1/1
  lbA/1 -> S-Function1/6
  ub/1 -> S-Function1/5
  lb/1 -> S-Function1/4
  ubA/1 -> S-Function1/7
  gradhT/1 -> S-Function1/3
  S-Function1/5 -> lambdaQP/1

== system NMPC/Nonlinear Model Predictive Engine Control/NMPC Algorithm/For Iterator Subsystem/NMPC Matrices/Hessian ==
  optVars : Inport
  p : Inport  Port=2
  lambda : Inport  Port=3
  Mux : Mux  Inputs=2
  Reshape1 : Reshape  OutputDimensionality=Customize  OutputDimensions=[parNMPC.nOptVars, parNMPC.nOptVars]
  S-Function : S-Function  FunctionName=sfun_qp_W  SFunctionDeploymentMode=off  EnableBusSupport=off
  W : Outport
  wires:
  Reshape1/1 -> W/1
  S-Function/1 -> Reshape1/1
  Mux/1 -> S-Function/2
  optVars/1 -> S-Function/1
  p/1 -> Mux/1
  lambda/1 -> Mux/2

== system NMPC/Nonlinear Model Predictive Engine Control/NMPC Algorithm/For Iterator Subsystem/NMPC Matrices/bA inequality ==
  optVars : Inport
  p : Inport  Port=2
  Reshape : Reshape  OutputDimensionality=Column vector (2-D)
  S-Function : S-Function  FunctionName=sfun_qp_h  SFunctionDeploymentMode=off  EnableBusSupport=off
  h : Outport
  wires:
  Reshape/1 -> h/1
  S-Function/1 -> Reshape/1
  p/1 -> S-Function/2
  optVars/1 -> S-Function/1

== system NMPC/Nonlinear Model Predictive Engine Control/NMPC Algorithm/For Iterator Subsystem/NMPC Matrices/grad hT matrix ==
  optVars : Inport
  p : Inport  Port=2
  Reshape1 : Reshape  OutputDimensionality=Customize  OutputDimensions=[parNMPC.nConstr,parNMPC.nOptVars]
  S-Function : S-Function  FunctionName=sfun_qp_gradhT  SFunctionDeploymentMode=off  EnableBusSupport=off
  gradhT : Outport
  wires:
  Reshape1/1 -> gradhT/1
  S-Function/1 -> Reshape1/1
  p/1 -> S-Function/2
  optVars/1 -> S-Function/1

== system NMPC/Nonlinear Model Predictive Engine Control/NMPC Algorithm/For Iterator Subsystem/NMPC Matrices/gradient ==
  optVars : Inport
  p : Inport  Port=2
  Reshape : Reshape  OutputDimensionality=Column vector (2-D)
  S-Function : S-Function  FunctionName=sfun_qp_gradJ  SFunctionDeploymentMode=off  EnableBusSupport=off
  gradJ : Outport
  wires:
  Reshape/1 -> gradJ/1
  optVars/1 -> S-Function/1
  p/1 -> S-Function/2
  S-Function/1 -> Reshape/1

== matlab function NMPC/Simulation Model/ROM/ROM/MATLAB Function ==
  data: xdot output; y output; x input; u input
function [xdot,y] = ROModel_Call(x,u)

%ROModel_Call: This function calls the reduced-order engine model to calculate
% the model outputs and all (continuous-time) derivatives of the model
% states, given the actual model inputs and model States.

[xdot,y] = ROModel(x,u);

end % function

% EOF

== matlab function NMPC/reference trajectory generator/MATLAB Function ==
  data: u input; y output size=[N,1]; N parameter size=1; Ts parameter double size=1
function y = fcn(u,N,Ts)

y = zeros(N,1);
y(1) = u;

for i=2:N
   y(i) = y(i-1)+Ts;
end


end

== matlab function NMPC/Nonlinear Model Predictive Engine Control/ROM/ROM/MATLAB Function ==
  data: xdot output; y output; x input; u input
function [xdot,y] = ROModel_Call(x,u)

%ROModel_Call: This function calls the reduced-order engine model to calculate
% the model outputs and all (continuous-time) derivatives of the model
% states, given the actual model inputs and model States.

[xdot,y] = ROModel(x,u);

end % function

% EOF

== matlab function NMPC/Nonlinear Model Predictive Engine Control/NMPC Algorithm/For Iterator Subsystem/NMPC Matrices/dL_calc ==
  data: lambda input; mu input; gradJ input; gradhT input; h input; normdL output size=1
function normdL = NormdLCalc(lambda,mu, gradJ,gradhT,h)

             normdL    = norm([gradJ - gradhT'*lambda + mu; h],2);

end

== matlab function NMPC/Nonlinear Model Predictive Engine Control/NMPC Algorithm/For Iterator Subsystem/stepSize_sk ==
  data: dvar input; dvarXalpha output size=parNMPC.N*(parNMPC.nStates + parNMPC.nInputs); alpha input size=1
function dvarXalpha  = product(dvar,alpha)

    dvarXalpha = dvar*alpha;

end

== matlab function NMPC/Nonlinear Model Predictive Engine Control/NMPC Algorithm/For Iterator Subsystem/Step Size Consideration lambda/stepSize_slambda_AOptVars ==
  data: slambda input; slambdaXalpha output; alpha input size=1
function slambdaXalpha  = product(slambda,alpha)

    slambdaXalpha = slambda*alpha;

end

== matlab function NMPC/Nonlinear Model Predictive Engine Control/NMPC Algorithm/For Iterator Subsystem/Step Size Consideration mu/stepSize_slambda_OptVars ==
  data: smu input; smuXalpha output; alpha input size=1
function smuXalpha  = product(smu,alpha)

    smuXalpha = smu*alpha;

end
